simulink library "common_lib"  (R2021b)
settings: Solver=ode45  StartTime=0.0  StopTime=10.0  RelTol=1e-3
undefined symbols (not defined in the file or in its folder): ACCEL_PRE_MULT, C_C1GearNumbers, C_C1GearRatios, C_Calibration, C_DitherWaveform, C_GearOffset, C_GearRatioIn, C_GearRatioInverseOut, C_GearRatioOut, CLUTCH_INNER_LOOP_UPDATE_RATE, CONSTANT, DEGRADED_MODE_SIZE, Dem_EventStatusType, DiscIntNeverNeededParam, F_FAULT_ENUM, F_NOFAULT, F_OUTOFRANGE, F_RATELIMIT, FALSE, FMI14_SPECIAL_INSTRUCTIONS, FMI20_DATA_DRIFTED_HIGH, FMI21_DATA_DRIFTED_LOW, FMI29_RESERVED_FOR_SAE_ASSIGNMENT, FMI30_RESERVED_FOR_SAE_ASSIGNMENT, FMI31_CONDITION_EXISTS, FMI32_NO_FAULT, IC, k_accel, k_mean, LVDCU_OORH_FaultCntThd_C, MAX_UINT32, MEAN_PRE_MULT, NTriggers, QLTY_SIGNAL_FAILED, QLTY_SIGNAL_FULLY_FUNCTION, QLTY_SIGNAL_SUBSTITUTED_BY_1ST_CHOICE, QLTY_SIGNAL_SUBSTITUTED_BY_2ND_CHOICE, QLTY_SIGNAL_SUBSTITUTED_BY_3RD_CHOICE, QLTY_SIGNAL_SUBSTITUTED_BY_4TH_CHOICE, SAMPLE_TIME_100_mSec, SAMPLE_TIME_100_uSec, simin, T_TestPoint, TF_FALSE, TF_TRUE, TimeStep, TRUE, WORKSPACE_UPDATE_RATE, ZERO, Zero
libraries: $bdroot x120, simulink x27, simulink_extras x4, MBD_EPS_Local_Blockset x4
(part 7 of 10)

== system common_lib/OS/fcn_call generator ==
  note: This component is an atomic element used by the
      | schedule_morph script to build scheduler blocks
  note: Common Library::OS::Function Call Generator
  Enable : EnablePort  StatesWhenEnabling=reset  ZeroCross=off
  Function-Call Generator : simulink/Ports & Subsystems/Function-Call Generator  sample_time=-1  numberOfIterations=1  DisallowWideOutput=off
  Out : Outport  VectorParamsAs1DForOutWhenUnconnected=off
  wires:
  Function-Call Generator/1 -> Out/1

== system common_lib/OS/schedule counter ==
  note: This component is an atomic element used by the
      | schedule_morph script to build scheduler blocks
  note: Common Library::OS::Schedule Counter
  Constant2 : Constant  Value=int8(1)
  Constant3 : Constant  Value=int8(1)
  Constant4 : Constant  Value=FALSE
  Constant5 : Constant  Value=int8(1)
  Logical Operator : Logic  Operator=OR
  MinMax1 : MinMax  Inputs=2  InputSameDT=on  ZeroCross=off
  NTriggers : Constant  Value=NTriggers
  Relational Operator1 : RelationalOperator  Operator=>  ZeroCross=off  RndMeth=Nearest
  Sum : Sum  Inputs=++|  InputSameDT=on  OutDataTypeStr=Inherit: Same as first input
  Sum1 : Sum  Inputs=|-+  InputSameDT=on  OutDataTypeStr=Inherit: Same as first input
  Unit Delay : UnitDelay  InitialCondition=int8(1)  SampleTime=-1  HasFrameUpgradeWarning=on
  Unit Delay1 : UnitDelay  InitialCondition=TRUE  SampleTime=-1  HasFrameUpgradeWarning=on
  reset switch : Switch  Threshold=0.5  ZeroCross=off  InputSameDT=on
  Counter : Outport  VectorParamsAs1DForOutWhenUnconnected=off
  wires:
  Constant5/1 -> Sum1/1
  Sum/1 -> MinMax1/2
  NTriggers/1 -> Sum1/2, MinMax1/1
  Sum1/1 -> Relational Operator1/2
  Relational Operator1/1 -> Logical Operator/1
  Constant3/1 -> reset switch/1
  MinMax1/1 -> reset switch/3
  Constant2/1 -> Sum/2
  Constant4/1 -> Unit Delay1/1
  Unit Delay1/1 -> Logical Operator/2
  Logical Operator/1 -> reset switch/2
  Unit Delay/1 -> Relational Operator1/1, Sum/1
  reset switch/1 -> Unit Delay/1, Counter/1

== system common_lib/OS/sequence generator ==
  note: This component is an atomic element used by the
      | schedule_morph script to build scheduler blocks
  note: Common Library::OS::Sequence Generator
  In : Inport
  Constant9 : Constant  Value=int8(1)
  Function-Call Generator : simulink/Ports & Subsystems/Function-Call Generator  sample_time=-1  numberOfIterations=1  DisallowWideOutput=off
  Sum1 : Sum  Inputs=|++  InputSameDT=on  OutDataTypeStr=Inherit: Same as first input
  Trigger : Outport  VectorParamsAs1DForOutWhenUnconnected=off
  Out : Outport  Port=2  VectorParamsAs1DForOutWhenUnconnected=off
  wires:
  Function-Call Generator/1 -> Trigger/1
  Constant9/1 -> Sum1/2
  In/1 -> Sum1/1
  Sum1/1 -> Out/1

== system common_lib/SCond/Gain and Offset (in) ==
  note: Common Library::Signal Conditioning::Gain and Offset (in)
  input : Inport
  gain : Inport  Port=2
  offset : Inport  Port=3
  InputConversion : DataTypeConversion  OutDataTypeStr=single  RndMeth=Zero
  InputConversion1 : DataTypeConversion  OutDataTypeStr=single  RndMeth=Zero
  InputConversion2 : DataTypeConversion  OutDataTypeStr=single  RndMeth=Zero
  OutputConversion : DataTypeConversion  OutDataTypeStr=single  RndMeth=Zero
  Product : Product  InputSameDT=on  OutDataTypeStr=Inherit: Same as first input
  Sum : Sum  Inputs=|+-  InputSameDT=on  OutDataTypeStr=Inherit: Same as first input
  output : Outport  VectorParamsAs1DForOutWhenUnconnected=off
  wires:
  OutputConversion/1 -> output/1
  input/1 -> InputConversion/1
  gain/1 -> InputConversion1/1
  Product/1 -> Sum/1
  offset/1 -> InputConversion2/1
  Sum/1 -> OutputConversion/1
  InputConversion/1 -> Product/1
  InputConversion1/1 -> Product/2
  InputConversion2/1 -> Sum/2

== system common_lib/SCond/Gain and Offset (out) ==
  note: Common Library::Signal Conditioning::Gain and Offset (out)
  input : Inport
  gain : Inport  Port=2
  offset : Inport  Port=3
  InputConversion : DataTypeConversion  OutDataTypeStr=single  RndMeth=Zero
  InputConversion1 : DataTypeConversion  OutDataTypeStr=single  RndMeth=Zero
  InputConversion2 : DataTypeConversion  OutDataTypeStr=single  RndMeth=Zero
  OutputConversion : DataTypeConversion  OutDataTypeStr=single  RndMeth=Zero
  Product : Product  Inputs=*/  InputSameDT=on  OutDataTypeStr=Inherit: Same as first input
  Sum : Sum  Inputs=|++  InputSameDT=on  OutDataTypeStr=Inherit: Same as first input
  output : Outport  VectorParamsAs1DForOutWhenUnconnected=off
  wires:
  Sum/1 -> Product/1
  input/1 -> InputConversion/1
  OutputConversion/1 -> output/1
  offset/1 -> InputConversion1/1
  gain/1 -> InputConversion2/1
  Product/1 -> OutputConversion/1
  InputConversion/1 -> Sum/1
  InputConversion1/1 -> Sum/2
  InputConversion2/1 -> Product/2

== system common_lib/SCond/Membership Function ==
  x : Inport
  Compare1 : RelationalOperator  Operator=<=  ZeroCross=off  RndMeth=Nearest  InputSameDT=on
  MinMax : MinMax  Function=max  Inputs=2  InputSameDT=on  SaturateOnIntegerOverflow=on  ZeroCross=off
  Product2 : Product  Inputs=**  OutDataTypeStr=Inherit: Same as first input
  Sum1 : Sum  Inputs=|++  InputSameDT=on  OutDataTypeStr=Inherit: Same as first input
  Sum2 : Sum  Inputs=-+|  InputSameDT=on  OutDataTypeStr=Inherit: Same as first input
  Switch1 : Switch  Criteria=u2 ~= 0  Threshold=0.5  ZeroCross=off  InputSameDT=on
  TRUE1 : Constant  Value=SlopeLow
  TRUE3 : Constant  Value=Peak
  TRUE4 : Constant  Value=One
  TRUE5 : Constant  Value=Zero
  TRUE6 : Constant  Value=SlopeHigh
  TRUE7 : Constant  Value=Peak
  mu(x) : Outport  VectorParamsAs1DForOutWhenUnconnected=off
  wires:
  Sum1/1 -> MinMax/2
  Switch1/1 -> Product2/2
  Product2/1 -> Sum1/1
  TRUE3/1 -> Compare1/2
  Compare1/1 -> Switch1/2
  TRUE6/1 -> Switch1/3
  TRUE1/1 -> Switch1/1
  Sum2/1 -> Product2/1
  TRUE7/1 -> Sum2/1
  x/1 -> Compare1/1, Sum2/2
  TRUE4/1 -> Sum1/2
  TRUE5/1 -> MinMax/1
  MinMax/1 -> mu(x)/1

== system common_lib/SCond/Test Override Gain and Offset (in) ==
  note: This block  accepts the Inputsignal, gain, offset, and override flag
      |
      | This block does the  functionality of Y =mX+b
      | Where  Y  = Output
      |               m = Override_Gain
      |               X  = Input
      |               b = Override_Offset
  note: Common Library::Signal Override::Gain , Offset ,Override flag
  Input : Inport
  Override_Gain : Inport  Port=2
  Override_Offset : Inport  Port=3
  Override_Flag : Inport  Port=4
  InputConversion : DataTypeConversion  OutDataTypeStr=single  RndMeth=Zero
  InputConversion1 : DataTypeConversion  OutDataTypeStr=single  RndMeth=Zero
  InputConversion2 : DataTypeConversion  OutDataTypeStr=single  RndMeth=Zero
  OutputConversion : DataTypeConversion  OutDataTypeStr=single  RndMeth=Zero
  Product : Product  InputSameDT=on  OutDataTypeStr=Inherit: Same as first input
  Sum : Sum  Inputs=|++  InputSameDT=on  OutDataTypeStr=Inherit: Same as first input
  Switch : Switch  Threshold=0.5  ZeroCross=off
  Output : Outport  VectorParamsAs1DForOutWhenUnconnected=off
  wires:
  InputConversion2/1 -> Sum/2
  InputConversion1/1 -> Product/2
  InputConversion/1 -> Product/1
  Sum/1 -> OutputConversion/1
  Product/1 -> Sum/1
  Input/1 -> InputConversion/1, Switch/3
  Switch/1 -> Output/1
  Override_Offset/1 -> InputConversion2/1
  Override_Flag/1 -> Switch/2
  Override_Gain/1 -> InputConversion1/1
  OutputConversion/1 -> Switch/1

== system common_lib/SCond/ramp to zero ==
  note: Common Library::Signal Conditioning::Ramp to Zero
  note: factor is zero at zero speed
      | factor is 1 or -1 if the abs value of spd is > limit
      | factor is linear between 1 and-1 if the abs value of spd < limit
      | the sign of factor is the same as the sign of speed
  speed : Inport
  limit : Inport  Port=2
  Abs : Abs  ZeroCross=off
  Constant : Constant  Value=One
  Constant1 : Constant  Value=MinusOne
  Constant2 : Constant  Value=Zero
  Product1 : Product  Inputs=*/  InputSameDT=on  OutDataTypeStr=Inherit: Same as first input
  Relational Operator : RelationalOperator  Operator=<  ZeroCross=off  RndMeth=Nearest  InputSameDT=on
  Relational Operator1 : RelationalOperator  ZeroCross=off  RndMeth=Nearest  InputSameDT=on
  Switch : Switch  Threshold=0.5  ZeroCross=off  InputSameDT=on
  Switch1 : Switch  Threshold=0.5  ZeroCross=off  InputSameDT=on
  factor : Outport  VectorParamsAs1DForOutWhenUnconnected=off
  wires:
  speed/1 -> Abs/1, Relational Operator1/1, Product1/1
  Abs/1 -> Relational Operator/1
  limit/1 -> Product1/2, Relational Operator/2
  Product1/1 -> Switch/1
  Relational Operator/1 -> Switch/2
  Constant/1 -> Switch1/1
  Switch/1 -> factor/1
  Constant1/1 -> Switch1/3
  Constant2/1 -> Relational Operator1/2
  Relational Operator1/1 -> Switch1/2
  Switch1/1 -> Switch/3

== system common_lib/Signal Conditioning/2nd Order Butterworth Filter ==
  note: DO NOT CHANGE 2.0 DAMPING CONSTANT
  note: This is a 2nd order butterworth filter.
      | When Disable is true the raw value is
      | passed through.
  note: The Integrator blocks in common_lib don't work as well
      | for this filter.
  Input : Inport
  CutoffFreq : Inport  Port=2
  Reset : Inport  Port=3
  ClampAboveZero : $bdroot/Misc/ClampAboveZero  Tol=single(0.001)
      settings: AttributesFormatString=tol=%<Tol>
  Constant1 : Constant  Value=single(0.0)  SampleTime=-1
  Constant2 : Constant  Value=single(2.0)  SampleTime=-1
  Constant3 : Constant  Value=TSAMP  SampleTime=-1
  Constant4 : Constant  Value=single(1.0)  SampleTime=-1
  Data Type Conversion : DataTypeConversion  OutDataTypeStr=single  RndMeth=Zero
  Divide : Product  Inputs=***
  Divide1 : Product  Inputs=***
  Divide2 : Product  Inputs=*/
  ForwardEulerIntergrator1 : MBD_EPS_Local_Blockset/Integrators/ForwardEulerIntergrator  IC=single(0.0)  TSAMP=TSAMP
  ForwardEulerIntergrator2 : MBD_EPS_Local_Blockset/Integrators/ForwardEulerIntergrator  IC=IC  TSAMP=TSAMP
  MinMax : MinMax  Inputs=2  InputSameDT=on  ZeroCross=off
  Sum : Sum  Inputs=|+-
  Sum1 : Sum  Inputs=|+-
  PtmShiftMotorTorqueCmd : Outport  VectorParamsAs1DForOutWhenUnconnected=off
  wires:
  Input/1 -> Sum/1, ForwardEulerIntergrator2/2
  Reset/1 -> ForwardEulerIntergrator2/3, ForwardEulerIntergrator1/3
  ForwardEulerIntergrator1/1 -> Divide1/3, ForwardEulerIntergrator2/1
  Sum1/1 -> ForwardEulerIntergrator1/1
  Divide1/1 -> Sum1/2
  Constant2/1 -> Divide1/2
  Sum/1 -> Divide/1
  ForwardEulerIntergrator2/1 -> PtmShiftMotorTorqueCmd/1, Sum/2
  Divide/1 -> Sum1/1
  Constant1/1 -> ForwardEulerIntergrator1/2
  CutoffFreq/1 -> MinMax/1
  Constant3/1 -> Data Type Conversion/1
  Constant4/1 -> Divide2/1
  Data Type Conversion/1 -> ClampAboveZero/1
  ClampAboveZero/1 -> Divide2/2
  Divide2/1 -> MinMax/2
  MinMax/1 -> [ProtectedCutoffFreq]
  [ProtectedCutoffFreq] -> Divide1/1, Divide/3, Divide/2

== system common_lib/Signal Conditioning/AnalogChecking ==
  in : Inport  OutDataTypeStr=Bus: BO_InputSignal
  u_lim : Inport  Port=2
  l_lim : Inport  Port=3
  r_lim : Inport  Port=4
  tau : Inport  Port=5
  overide : Inport  Port=6
  overide_value : Inport  Port=7
  Bitwise Operator : simulink/Logic and Bit Operations/Bitwise Operator  logicop=OR  UseBitMask=off  NumInputPorts=3  BitMask=bin2dec('11011001')  BitMaskRealWorld=Stored Integer
  Bus Creator2 : BusCreator  Inputs=2  OutDataTypeStr=Bus: BO_InputSignal
  Bus Selector1 : BusSelector  OutputSignals=value,FMI
  C_Calibration1 : Constant  Value=F_OUTOFRANGE
  C_Calibration2 : Constant  Value=F_NOFAULT
  C_Calibration3 : Constant  Value=false
  C_Calibration4 : Constant  Value=F_RATELIMIT
  C_Calibration5 : Constant  Value=F_NOFAULT
  C_Calibration6 : Constant  Value=false
  C_Calibration7 : Constant  Value=F_NOFAULT
  C_Calibration8 : Constant  Value=false
  Fltr_wR : $bdroot/Fltrs/Fltr_wR  TimeStep=TimeStep
  Logical Operator : Logic  Operator=OR
  OOR Fault Detection : $bdroot/Diag/OOR Fault Detection  InitialValue=0
  Rate Limit Fault Detection : $bdroot/Diag/Rate Limit Fault Detection  IC=0  TimeStep=TimeStep
  Relational Operator : RelationalOperator  Operator=~=  OutDataTypeStr=boolean  ZeroCross=off  RndMeth=Nearest
  Switch : Switch  Threshold=0.5  ZeroCross=off
  Switch1 : Switch  Threshold=0.5  ZeroCross=off
  Switch2 : Switch  Threshold=0.5  ZeroCross=off
  Unit Delay : UnitDelay  InitialCondition=true  SampleTime=-1  HasFrameUpgradeWarning=on
      settings: AttributesFormatString=ic=%<X0>
  out : Outport  VectorParamsAs1DForOutWhenUnconnected=off
  wires:
  Relational Operator/1 -> Logical Operator/2
  Logical Operator/1 -> Fltr_wR/4
  Unit Delay/1 -> Logical Operator/1
  C_Calibration8/1 -> Unit Delay/1
  Bus Selector1/1 -> OOR Fault Detection/1  "<value>"
  C_Calibration6/1 -> OOR Fault Detection/4
  in/1 -> Bus Selector1/1
  OOR Fault Detection/1 -> Rate Limit Fault Detection/1
  u_lim/1 -> OOR Fault Detection/2
  l_lim/1 -> OOR Fault Detection/3
  Bus Selector1/2 -> Bitwise Operator/3  "<FMI>"
  OOR Fault Detection/2 -> Switch/2
  Switch/1 -> Bitwise Operator/2
  C_Calibration1/1 -> Switch/1
  C_Calibration2/1 -> Switch/3
  Bus Creator2/1 -> out/1
  Rate Limit Fault Detection/1 -> Fltr_wR/3, Fltr_wR/1
  r_lim/1 -> Rate Limit Fault Detection/2
  C_Calibration3/1 -> Rate Limit Fault Detection/3
  Rate Limit Fault Detection/2 -> Switch1/2
  C_Calibration4/1 -> Switch1/1
  C_Calibration5/1 -> Switch1/3
  Switch1/1 -> Bitwise Operator/1
  Bitwise Operator/1 -> Bus Creator2/2, Relational Operator/2  "FMI"
  tau/1 -> Fltr_wR/2
  C_Calibration7/1 -> Relational Operator/1
  overide/1 -> Switch2/2
  overide_value/1 -> Switch2/1
  Fltr_wR/1 -> Switch2/3  "value"
  Switch2/1 -> Bus Creator2/1  "value"

== system common_lib/Signal Conditioning/DitherSaturation ==
  signal_in : Inport
  max_signal_amp : Inport  Port=2
  dither_amplitude : Inport  Port=3
  dither_in : Inport  Port=4
  Constant1 : Constant  Value=0  OutDataTypeStr=single
  Constant2 : Constant  Value=single(1)
  Constant3 : Constant  Value=eps  OutDataTypeStr=single
  MinMax1 : MinMax  Inputs=2
  MinMax2 : MinMax  Inputs=2
  MinMax3 : MinMax  Function=max  Inputs=2
  MinMax4 : MinMax  Inputs=2
  MinMax5 : MinMax  Function=max  Inputs=2
  Product : Product  RndMeth=Zero
  Product1 : Product  RndMeth=Zero
  Product2 : Product  Inputs=/*  RndMeth=Zero
  Product3 : Product  Inputs=/*  RndMeth=Zero
  Sum : Sum  Inputs=|-+
  Sum1 : Sum  Inputs=|++
  out : Outport  VectorParamsAs1DForOutWhenUnconnected=off
  wires:
  Constant1/1 -> MinMax5/2
  signal_in/1 -> MinMax5/1
  MinMax5/1 -> MinMax4/2
  MinMax4/1 -> Product2/2, Sum/1, Sum1/2
  Product1/1 -> Sum1/1
  Sum1/1 -> out/1
  dither_in/1 -> Product/1
  MinMax3/1 -> Product2/1, Product3/1
  Constant3/1 -> MinMax3/2
  Product/1 -> Product1/1
  Product3/1 -> MinMax1/2
  Sum/1 -> Product3/2
  Product2/1 -> MinMax1/1
  MinMax2/1 -> Product1/2
  MinMax1/1 -> MinMax2/2
  Constant2/1 -> MinMax2/1
  max_signal_amp/1 -> MinMax4/1, Sum/2
  dither_amplitude/1 -> Product/2, MinMax3/1

== system common_lib/Signal Conditioning/DitherSaturation1 ==
  signal_in : Inport
  max_signal_amp : Inport  Port=2
  dither_amplitude : Inport  Port=3
  dither_in : Inport  Port=4
  Constant1 : Constant  Value=0  OutDataTypeStr=single
  Constant2 : Constant  Value=single(1)
  Constant3 : Constant  Value=eps  OutDataTypeStr=single
  MinMax1 : MinMax  Inputs=2
  MinMax2 : MinMax  Inputs=2
  MinMax3 : MinMax  Function=max  Inputs=2
  MinMax4 : MinMax  Inputs=2
  MinMax5 : MinMax  Function=max  Inputs=2
  Product : Product  RndMeth=Zero
  Product1 : Product  RndMeth=Zero
  Product2 : Product  Inputs=/*  RndMeth=Zero
  Product3 : Product  Inputs=/*  RndMeth=Zero
  Sum : Sum  Inputs=|-+
  Sum1 : Sum  Inputs=|++
  out : Outport  VectorParamsAs1DForOutWhenUnconnected=off
  wires:
  Constant1/1 -> MinMax5/2
  signal_in/1 -> MinMax5/1
  MinMax5/1 -> MinMax4/2
  MinMax4/1 -> Product2/2, Sum/1, Sum1/2
  Product1/1 -> Sum1/1
  Sum1/1 -> out/1
  dither_in/1 -> Product/1
  MinMax3/1 -> Product2/1, Product3/1
  Constant3/1 -> MinMax3/2
  Product/1 -> Product1/1
  Product3/1 -> MinMax1/2
  Sum/1 -> Product3/2
  Product2/1 -> MinMax1/1
  MinMax2/1 -> Product1/2
  MinMax1/1 -> MinMax2/2
  Constant2/1 -> MinMax2/1
  max_signal_amp/1 -> MinMax4/1, Sum/2
  dither_amplitude/1 -> Product/2, MinMax3/1

== system common_lib/Signal Conditioning/HydValveDither ==
  freq_hz : Inport
  CalculateActualFreq : Subsystem
  Constant : Constant  Value=single(ts)
  Constant4 : Constant  Value=single(0)
  Switch : Switch  Criteria=u2 > Threshold
  TableBasedSignalGen : Subsystem
  out : Outport  VectorParamsAs1DForOutWhenUnconnected=off
  realized_freq : Outport  Port=2  VectorParamsAs1DForOutWhenUnconnected=off
  wires:
  Constant4/1 -> Switch/3
  TableBasedSignalGen/1(out) -> Switch/1
  freq_hz/1 -> CalculateActualFreq/1(desired_freqency_hz), Switch/2
  CalculateActualFreq/2(sample_times_per_cycle) -> TableBasedSignalGen/1(sample_times_per_cycle)
  CalculateActualFreq/1(realized_freq) -> realized_freq/1
  Constant/1 -> CalculateActualFreq/2(sample_time)
  Switch/1 -> out/1

== system common_lib/Signal Conditioning/Normalized Variable Tanh Curve ==
  note: Time Input
  note: This block handles a changing Target Time
  note: ******************************************************************************************************************************************************
      | UNPUBLISHED AND CONFIDENTIAL. COPYRIGHT EATON CORPORATION, CREATED 2002, ALL RIGHTS RESERVED.
      | NOT TO BE REPRODUCED, DISSEMINATED, TRANSFERRED OR USED WITHOUT THE PRIOR WRITTEN CONSENT OF
      | EATON CORPORATION.
      | ******************************************************************************************************************************************************
  RampTime : Inport
  Reset : Inport  Port=2
  ClampAboveZero : $bdroot/Misc/ClampAboveZero  Tol=single(0.001)
      settings: AttributesFormatString=tol=%<Tol>
  Constant12 : Constant  Value=single(1000)  SampleTime=-1
  Constant13 : Constant  Value=single(-1000)  SampleTime=-1
  Constant3 : Constant  Value=TimeStep  SampleTime=-1
  Constant7 : Constant  Value=single(0)  SampleTime=-1
  Constant8 : Constant  Value=single(-1000)  SampleTime=-1
  Constant9 : Constant  Value=single(0.0)  SampleTime=-1
  Data Type Conversion : DataTypeConversion  OutDataTypeStr=single  RndMeth=Zero
  Lookup Table Tanh : Lookup  InputValues=single([0 0.125 0.25 0.375 0.5 0.625 0.75 0.875 1])  Table=single([0 0.04745 0.1192 0.26895 0.5 0.73105 0.8808 0.95255 1])  LookUpMeth=Interpolation-Use End Values
  Product1 : Product  Inputs=*/  OutDataTypeStr=Inherit: Same as first input
  Sum1 : Sum  Inputs=|++
  Switch : Switch  Threshold=0.5  ZeroCross=off
  Trajectory : MBD_EPS_Local_Blockset/Trajectory Modification/Trajectory  TimeStep=TimeStep  wn=single(30)  damping=single(.8)
  Unit Delay : UnitDelay  InitialCondition=single(0.0)  SampleTime=-1  HasFrameUpgradeWarning=on
      settings: AttributesFormatString=ic=%<X0>
  Out : Outport  VectorParamsAs1DForOutWhenUnconnected=off
  wires:
  Product1/1 -> Lookup Table Tanh/1
  Unit Delay/1 -> Sum1/2
  Constant3/1 -> Data Type Conversion/1
  Constant7/1 -> Trajectory/2
  Lookup Table Tanh/1 -> Out/1
  Trajectory/1 -> ClampAboveZero/1
  RampTime/1 -> Trajectory/1
  Constant8/1 -> Trajectory/3
  Constant12/1 -> Trajectory/4
  Constant13/1 -> Trajectory/5
  Reset/1 -> Switch/2, Trajectory/6
  Constant9/1 -> Switch/1
  Sum1/1 -> Switch/3
  Switch/1 -> Unit Delay/1, Product1/1
  ClampAboveZero/1 -> Product1/2
  Data Type Conversion/1 -> Sum1/1

== system common_lib/Signal Conditioning/Obsolete Signal Conditioning ==
  note: Obsolete Signal Conditioning
  BooleanToTernary : Subsystem
      mask Display:
      | patch([0.3 0.3 0.7 0.7], [0.4 0.6 0.6 0.4], [255/255 127/255 255/255]);
      | disp('Boolean to Ternary')
  Ternary To Boolean (Default False) : Subsystem
      mask Display:
      | patch([0.3 0.3 0.7 0.7], [0.4 0.6 0.6 0.4], [255/255 127/255 255/255]);
      | disp('Ternary To Boolean\n(Default False)')
  Ternary To Boolean (Default True) : Subsystem
      mask Display:
      | patch([0.3 0.3 0.7 0.7], [0.4 0.6 0.6 0.4], [255/255 127/255 255/255]);
      | disp('Ternary To Boolean \n (Default True)')

== system common_lib/Signal Conditioning/OffsetAndGain ==
  input : Inport
  gain : Inport  Port=2
  offset : Inport  Port=3
  Data Type Conversion : DataTypeConversion  OutDataTypeStr=single
  Data Type Conversion1 : DataTypeConversion  OutDataTypeStr=single
  Data Type Conversion2 : DataTypeConversion  OutDataTypeStr=single
  Product : Product  InputSameDT=on  OutDataTypeStr=Inherit: Same as first input
  Sum : Sum  InputSameDT=on  OutDataTypeStr=Inherit: Same as first input
  output : Outport  VectorParamsAs1DForOutWhenUnconnected=off
  wires:
  Data Type Conversion2/1 -> Product/2
  Data Type Conversion1/1 -> Sum/2
  Data Type Conversion/1 -> Sum/1
  Sum/1 -> Product/1
  Product/1 -> output/1
  offset/1 -> Data Type Conversion/1
  gain/1 -> Data Type Conversion2/1
  input/1 -> Data Type Conversion1/1

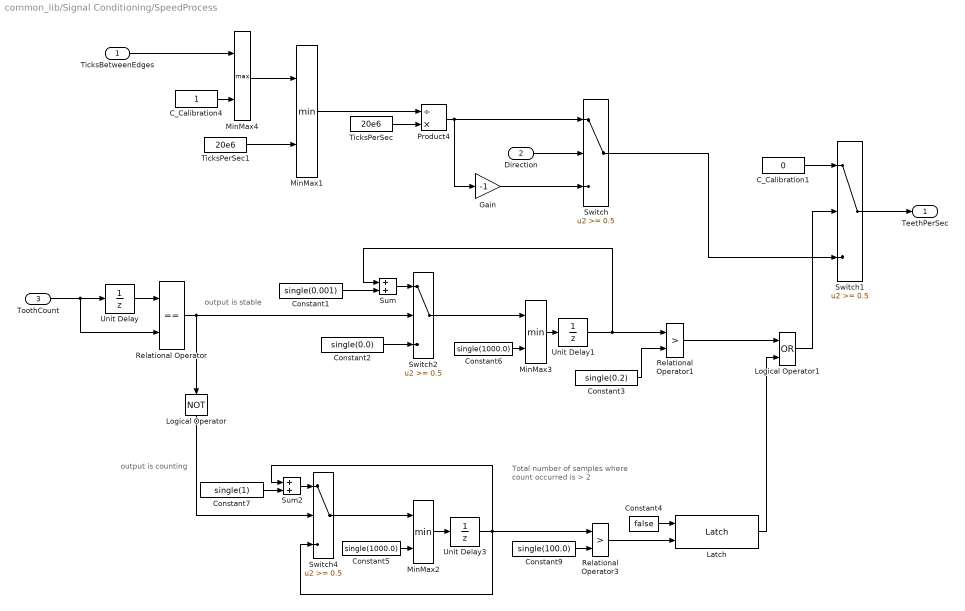
== system common_lib/Signal Conditioning/SpeedProcess ==
  note: output is stable
  note: output is counting
  note: Total number of samples where
      | count occurred is > 2
  TicksBetweenEdges : Inport
  Direction : Inport  Port=2
  ToothCount : Inport  Port=3
  C_Calibration1 : Constant  Value=0
  C_Calibration4 : Constant
  Constant1 : Constant  Value=single(0.001)
  Constant2 : Constant  Value=single(0.0)
  Constant3 : Constant  Value=single(0.2)
  Constant4 : Constant  Value=false
  Constant5 : Constant  Value=single(1000.0)
  Constant6 : Constant  Value=single(1000.0)
  Constant7 : Constant  Value=single(1)
  Constant9 : Constant  Value=single(100.0)
  Gain : Gain  Gain=-1
  Latch : $bdroot/Misc/Latch  IC=true
  Logical Operator : Logic  Operator=NOT
  Logical Operator1 : Logic  Operator=OR  AllPortsSameDT=off
  MinMax1 : MinMax  Inputs=2  InputSameDT=on  ZeroCross=off
  MinMax2 : MinMax  Inputs=2  InputSameDT=on  ZeroCross=off
  MinMax3 : MinMax  Inputs=2  InputSameDT=on  ZeroCross=off
  MinMax4 : MinMax  Function=max  Inputs=2  InputSameDT=on  ZeroCross=off
  Product4 : Product  Inputs=/*  RndMeth=Zero
  Relational Operator : RelationalOperator  Operator===  OutDataTypeStr=boolean  RndMeth=Nearest
  Relational Operator1 : RelationalOperator  Operator=>  ZeroCross=off  RndMeth=Nearest
  Relational Operator3 : RelationalOperator  Operator=>  ZeroCross=off  RndMeth=Nearest
  Sum : Sum
  Sum2 : Sum
  Switch{,1..2,4} (4 alike) : Switch  Threshold=0.5  ZeroCross=off
  TicksPerSec : Constant  Value=20e6
  TicksPerSec1 : Constant  Value=20e6
  Unit Delay : UnitDelay  SampleTime=0.001  HasFrameUpgradeWarning=on
  Unit Delay1 : UnitDelay  InitialCondition=single(0)  SampleTime=0.001  HasFrameUpgradeWarning=on
  Unit Delay3 : UnitDelay  InitialCondition=single(0)  SampleTime=0.001  HasFrameUpgradeWarning=on
  TeethPerSec : Outport  VectorParamsAs1DForOutWhenUnconnected=off
  wires:
  Constant3/1 -> Relational Operator1/2
  Constant2/1 -> Switch2/3
  Unit Delay1/1 -> Relational Operator1/1, Sum/1
  MinMax1/1 -> Product4/1
  TicksPerSec1/1 -> MinMax1/2
  MinMax4/1 -> MinMax1/1
  Switch1/1 -> TeethPerSec/1
  TicksPerSec/1 -> Product4/2
  TicksBetweenEdges/1 -> MinMax4/1
  Direction/1 -> Switch/2
  Gain/1 -> Switch/3
  Product4/1 -> Gain/1, Switch/1
  ToothCount/1 -> Unit Delay/1, Relational Operator/2
  C_Calibration4/1 -> MinMax4/2
  Unit Delay/1 -> Relational Operator/1
  Sum/1 -> Switch2/1
  Constant1/1 -> Sum/2
  Relational Operator/1 -> Switch2/2, Logical Operator/1
  C_Calibration1/1 -> Switch1/1
  Switch/1 -> Switch1/3
  Logical Operator/1 -> Switch4/2
  Constant9/1 -> Relational Operator3/2
  Unit Delay3/1 -> Sum2/1, Switch4/3, Relational Operator3/1
  Sum2/1 -> Switch4/1
  Constant7/1 -> Sum2/2
  Latch/1 -> Logical Operator1/2
  Relational Operator3/1 -> Latch/2
  Constant4/1 -> Latch/1
  Relational Operator1/1 -> Logical Operator1/1
  Logical Operator1/1 -> Switch1/2
  MinMax2/1 -> Unit Delay3/1
  Switch4/1 -> MinMax2/1
  Constant5/1 -> MinMax2/2
  MinMax3/1 -> Unit Delay1/1
  Constant6/1 -> MinMax3/2
  Switch2/1 -> MinMax3/1

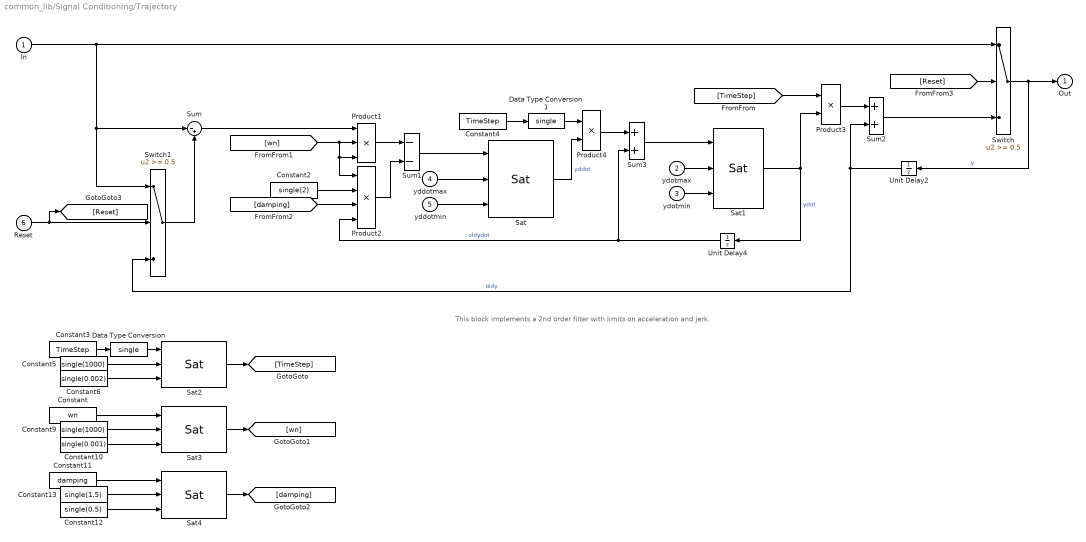
== system common_lib/Signal Conditioning/Trajectory ==
  note: This block implements a 2nd order filter with limits on acceleration and jerk.
  In : Inport
  ydotmax : Inport  Port=2
  ydotmin : Inport  Port=3
  yddotmax : Inport  Port=4
  yddotmin : Inport  Port=5
  Reset : Inport  Port=6
  Constant : Constant  Value=wn  SampleTime=-1
  Constant10 : Constant  Value=single(0.001)  SampleTime=-1
  Constant11 : Constant  Value=damping  SampleTime=-1
  Constant12 : Constant  Value=single(0.5)  SampleTime=-1
  Constant13 : Constant  Value=single(1.5)  SampleTime=-1
  Constant2 : Constant  Value=single(2)  SampleTime=-1
  Constant3 : Constant  Value=TimeStep  SampleTime=-1
  Constant4 : Constant  Value=TimeStep  SampleTime=-1
  Constant5 : Constant  Value=single(1000)  SampleTime=-1
  Constant6 : Constant  Value=single(0.002)  SampleTime=-1
  Constant9 : Constant  Value=single(1000)  SampleTime=-1
  Data Type Conversion : DataTypeConversion  OutDataTypeStr=single  RndMeth=Zero
  Data Type Conversion1 : DataTypeConversion  OutDataTypeStr=single  RndMeth=Zero
  Product1 : Product  Inputs=3  OutDataTypeStr=Inherit: Same as first input
  Product2 : Product  Inputs=4  OutDataTypeStr=Inherit: Same as first input
  Product3 : Product  OutDataTypeStr=Inherit: Same as first input
  Product4 : Product  OutDataTypeStr=Inherit: Same as first input
  Sat{,1..4} (5 alike) : $bdroot/Slink/Sat
  Sum : Sum  Inputs=|-+
  Sum1 : Sum  Inputs=--
  Sum2 : Sum
  Sum3 : Sum
  Switch : Switch  Threshold=0.5  ZeroCross=off
  Switch1 : Switch  Threshold=0.5  ZeroCross=off
  Unit Delay2 : UnitDelay  InitialCondition=single(0.0)  SampleTime=-1  HasFrameUpgradeWarning=on
      settings: AttributesFormatString=ic=%<X0>
  Unit Delay4 : UnitDelay  InitialCondition=single(0.0)  SampleTime=-1  HasFrameUpgradeWarning=on
      settings: AttributesFormatString=ic=%<X0>
  Out : Outport  VectorParamsAs1DForOutWhenUnconnected=off
  wires:
  In/1 -> Switch/1, Switch1/1, Sum/1
  Sum/1 -> Product1/1
  Product2/1 -> Sum1/2
  Product1/1 -> Sum1/1
  Product3/1 -> Sum2/1
  Constant4/1 -> Data Type Conversion1/1
  Product4/1 -> Sum3/1
  Sum3/1 -> Sat1/1
  Constant2/1 -> Product2/2
  Sum1/1 -> Sat/1
  yddotmax/1 -> Sat/2
  yddotmin/1 -> Sat/3
  Sat/1 -> Product4/2  "yddot"
  ydotmax/1 -> Sat1/2
  Sat1/1 -> Unit Delay4/1, Product3/2  "ydot"
  Switch/1 -> Out/1, Unit Delay2/1  "y"
  Sum2/1 -> Switch/3
  Unit Delay2/1 -> Sum2/2, Switch1/3  "oldy"
  Unit Delay4/1 -> Sum3/2, Product2/4  "oldydot"
  Switch1/1 -> Sum/2
  ydotmin/1 -> Sat1/3
  Constant3/1 -> Data Type Conversion/1
  Constant5/1 -> Sat2/2
  Constant6/1 -> Sat2/3
  Sat2/1 -> [TimeStep]
  [TimeStep] -> Product3/1
  Constant/1 -> Sat3/1
  Constant9/1 -> Sat3/2
  Constant10/1 -> Sat3/3
  Sat3/1 -> [wn]
  [wn] -> Product1/2, Product1/3, Product2/1
  Constant11/1 -> Sat4/1
  Constant13/1 -> Sat4/2
  Constant12/1 -> Sat4/3
  Sat4/1 -> [damping]
  [damping] -> Product2/3
  Reset/1 -> Switch1/2, [Reset]
  [Reset] -> Switch/2
  Data Type Conversion/1 -> Sat2/1
  Data Type Conversion1/1 -> Product4/1

== system common_lib/Signal Conditioning/Variable Tanh Curve ==
  note: ******************************************************************************************************************************************************
      | UNPUBLISHED AND CONFIDENTIAL. COPYRIGHT EATON CORPORATION, CREATED 2002, ALL RIGHTS RESERVED.
      | NOT TO BE REPRODUCED, DISSEMINATED, TRANSFERRED OR USED WITHOUT THE PRIOR WRITTEN CONSENT OF
      | EATON CORPORATION.
      | ******************************************************************************************************************************************************
  StartValue : Inport
  FinalValue : Inport  Port=2
  RampTime : Inport  Port=3
  Reset : Inport  Port=4
  Constant1 : Constant  Value=single(0.01)  SampleTime=-1
  Constant10 : Constant  Value=single(1.0)  SampleTime=-1
  Normalized Variable Tanh Curve : MBD_EPS_Local_Blockset/Trajectory Modification/Normalized Variable Tanh Curve  TimeStep=TimeStep
  Product2 : Product  OutDataTypeStr=Inherit: Same as first input
  Relational Operator : RelationalOperator  Operator=<=  ZeroCross=off  RndMeth=Nearest
  Sum2 : Sum  Inputs=|+-
  Sum5 : Sum  Inputs=|+-
  Sum6 : Sum  Inputs=+-|
  Switch : Switch  Threshold=0.5  ZeroCross=off
  Unit Delay1 : UnitDelay  InitialCondition=single(0.0)  SampleTime=-1  HasFrameUpgradeWarning=on
      settings: AttributesFormatString=ic=%<X0>
  Out : Outport  VectorParamsAs1DForOutWhenUnconnected=off
  RampComplete : Outport  Port=2  VectorParamsAs1DForOutWhenUnconnected=off
  wires:
  RampTime/1 -> Normalized Variable Tanh Curve/1
  FinalValue/1 -> Sum5/1, Sum6/1
  StartValue/1 -> Switch/1
  Switch/1 -> Unit Delay1/1, Sum6/2
  Unit Delay1/1 -> Switch/3
  Constant10/1 -> Sum2/1
  Normalized Variable Tanh Curve/1 -> Sum2/2
  Sum6/1 -> Product2/1
  Sum2/1 -> Product2/2, Relational Operator/1
  Product2/1 -> Sum5/2
  Sum5/1 -> Out/1
  Constant1/1 -> Relational Operator/2
  Relational Operator/1 -> RampComplete/1
  Reset/1 -> Switch/2, Normalized Variable Tanh Curve/2

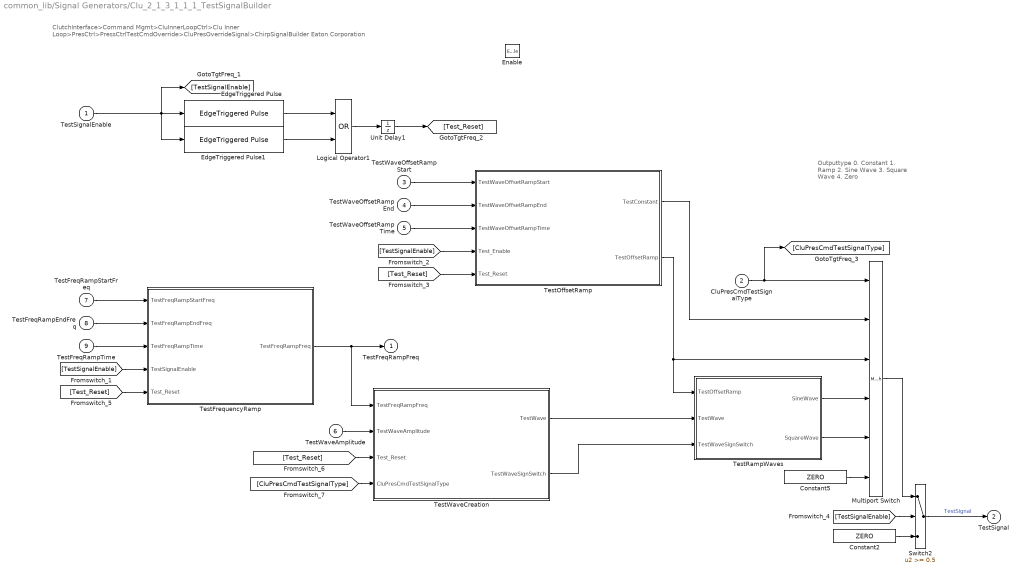
== system common_lib/Signal Generators/Clu_2_1_3_1_1_1_TestSignalBuilder ==
  note: ClutchInterface>Command Mgmt>CluInnerLoopCtrl>Clu Inner Loop>PresCtrl>PressCtrlTestCmdOverride>CluPresOverrideSignal>ChirpSignalBuilder
      | Eaton Corporation
  note: Outputtype
      | 0. Constant
      | 1. Ramp
      | 2. Sine Wave
      | 3. Square Wave
      | 4. Zero
  TestSignalEnable : Inport
  CluPresCmdTestSignalType : Inport  Port=2
  TestWaveOffsetRampStart : Inport  Port=3
  TestWaveOffsetRampEnd : Inport  Port=4
  TestWaveOffsetRampTime : Inport  Port=5
  TestWaveAmplitude : Inport  Port=6
  TestFreqRampStartFreq : Inport  Port=7
  TestFreqRampEndFreq : Inport  Port=8
  TestFreqRampTime : Inport  Port=9
  Enable : EnablePort  ZeroCross=off
  Constant2 : Constant  Value=ZERO
  Constant5 : Constant  Value=ZERO
  EdgeTriggered Pulse : $bdroot/Misc/EdgeTriggered Pulse  Edge=FALSE to TRUE  Width=single(0.01)  Pulse=TRUE  TimeStep=CLUTCH_INNER_LOOP_UPDATE_RATE  Init=0
  EdgeTriggered Pulse1 : $bdroot/Misc/EdgeTriggered Pulse  Edge=TRUE to FALSE  Width=single(0.01)  Pulse=TRUE  TimeStep=CLUTCH_INNER_LOOP_UPDATE_RATE  Init=0
  Logical Operator1 : Logic  Operator=OR  AllPortsSameDT=off
  Multiport Switch : MultiPortSwitch  DataPortOrder=Zero-based contiguous  Inputs=4  DataPortForDefault=Additional data port  zeroidx=on
  Switch2 : Switch  Threshold=0.5  ZeroCross=off
  TestFrequencyRamp : Subsystem
  TestOffsetRamp : Subsystem
  TestRampWaves : Subsystem
  TestWaveCreation : Subsystem
  Unit Delay1 : UnitDelay  InitialCondition=true  SampleTime=-1  HasFrameUpgradeWarning=on
      settings: AttributesFormatString=ic=%<X0>
  TestFreqRampFreq : Outport  InitialOutput=[single(0)]  VectorParamsAs1DForOutWhenUnconnected=off
      settings: AttributesFormatString=InitialOutput=%<InitialOutput>\nOutputWhenDisabled=%<OutputWhenDisabled>
  TestSignal : Outport  Port=2  InitialOutput=[single(0)]  VectorParamsAs1DForOutWhenUnconnected=off
      settings: AttributesFormatString=InitialOutput=%<InitialOutput>\nOutputWhenDisabled=%<OutputWhenDisabled>
  wires:
  TestOffsetRamp/2(TestOffsetRamp) -> TestRampWaves/1(TestOffsetRamp), Multiport Switch/3
  Constant5/1 -> Multiport Switch/6
  Multiport Switch/1 -> Switch2/1
  CluPresCmdTestSignalType/1 -> Multiport Switch/1, [CluPresCmdTestSignalType]
  Switch2/1 -> TestSignal/1  "TestSignal"
  Constant2/1 -> Switch2/3
  TestFrequencyRamp/1(TestFreqRampFreq) -> TestFreqRampFreq/1, TestWaveCreation/1(TestFreqRampFreq)
  Logical Operator1/1 -> Unit Delay1/1
  EdgeTriggered Pulse/1 -> Logical Operator1/1
  EdgeTriggered Pulse1/1 -> Logical Operator1/2
  TestSignalEnable/1 -> EdgeTriggered Pulse/1, EdgeTriggered Pulse1/1, [TestSignalEnable]
  Unit Delay1/1 -> [Test_Reset]
  [TestSignalEnable] -> TestFrequencyRamp/4(TestSignalEnable)
  TestFreqRampEndFreq/1 -> TestFrequencyRamp/2(TestFreqRampEndFreq)
  TestFreqRampStartFreq/1 -> TestFrequencyRamp/1(TestFreqRampStartFreq)
  TestFreqRampTime/1 -> TestFrequencyRamp/3(TestFreqRampTime)
  [Test_Reset] -> TestFrequencyRamp/5(Test_Reset)
  TestWaveAmplitude/1 -> TestWaveCreation/2(TestWaveAmplitude)
  [TestSignalEnable] -> TestOffsetRamp/4(Test_Enable)
  [Test_Reset] -> TestOffsetRamp/5(Test_Reset)
  TestWaveOffsetRampTime/1 -> TestOffsetRamp/3(TestWaveOffsetRampTime)
  TestWaveOffsetRampStart/1 -> TestOffsetRamp/1(TestWaveOffsetRampStart)
  TestWaveOffsetRampEnd/1 -> TestOffsetRamp/2(TestWaveOffsetRampEnd)
  TestOffsetRamp/1(TestConstant) -> Multiport Switch/2
  TestWaveCreation/1(TestWave) -> TestRampWaves/2(TestWave)
  [TestSignalEnable] -> Switch2/2
  [Test_Reset] -> TestWaveCreation/3(Test_Reset)
  [CluPresCmdTestSignalType] -> TestWaveCreation/4(CluPresCmdTestSignalType)
  TestWaveCreation/2(TestWaveSignSwitch) -> TestRampWaves/3(TestWaveSignSwitch)
  TestRampWaves/1(SineWave) -> Multiport Switch/4
  TestRampWaves/2(SquareWave) -> Multiport Switch/5

== system common_lib/Signal Generators/CustomProfileGenerator ==
  CustomProfileTimeVector : Inport
  CustomProfileOutputVector : Inport  Port=2
  CustomProfileRepeat : Inport  Port=3
  TestSignalReset : Inport  Port=4
  2D Lookup : $bdroot/Tbl/2D Lookup  Mode=Linear Interpolation
  Constant1 : Constant  Value=single(0.0)
  Logical Operator : Logic  Operator=OR  AllPortsSameDT=off
  Logical Operator1 : Logic  AllPortsSameDT=off
  MinMax : MinMax  Function=max  InputSameDT=on  ZeroCross=off
  Relational Operator : RelationalOperator  ZeroCross=off  RndMeth=Nearest
  Switch1 : Switch  Threshold=0.5  ZeroCross=off
  TestSignalTimer : $bdroot/Signal Generators/Signal Generator Components/TestSignalTimer  TimeStep=TimeStep
  Unit Delay5 : UnitDelay  InitialCondition=single(0.0)  SampleTime=-1  HasFrameUpgradeWarning=on
      settings: AttributesFormatString=ic=%<X0>
  CustomProfileOutput : Outport  VectorParamsAs1DForOutWhenUnconnected=off
  wires:
  TestSignalReset/1 -> [TestSignalReset], Logical Operator/1
  TestSignalTimer/1 -> [TestSignalTime]
  [TestSignalTime] -> 2D Lookup/1
  CustomProfileTimeVector/1 -> 2D Lookup/2, MinMax/1
  CustomProfileOutputVector/1 -> 2D Lookup/3
  MinMax/1 -> Relational Operator/2
  [TestSignalTime] -> Unit Delay5/1
  Unit Delay5/1 -> Relational Operator/1
  Relational Operator/1 -> Logical Operator1/2
  Logical Operator/1 -> TestSignalTimer/1
  CustomProfileRepeat/1 -> Logical Operator1/1
  Logical Operator1/1 -> Logical Operator/2
  Constant1/1 -> Switch1/1
  2D Lookup/1 -> Switch1/3
  [TestSignalReset] -> Switch1/2
  Switch1/1 -> CustomProfileOutput/1

== system common_lib/Signal Generators/Signal Generator Components ==
  note: Signal Generator Components
  TestSignalPeriod : Subsystem  mask{TimeStep=TimeStep}
      mask prompts: TimeStep "Time Step"
  TestSignalPeriodTimer : Subsystem  mask{TimeStep=TimeStep}
      mask prompts: TimeStep "Time Step"
  TestSignalRamp : Subsystem  mask{TimeStep=TimeStep}
      mask prompts: TimeStep "Time Step"
  TestSignalSineWave : Subsystem
  TestSignalSquareTriangleWave_Advanced : Subsystem  mask{TimeStep=TimeStep}
      mask prompts: TimeStep "Time Step"
  TestSignalSquareTriangleWave_Basic : Subsystem  mask{TimeStep=TimeStep}
      mask prompts: TimeStep "Time Step"
  TestSignalTimer : Subsystem  mask{TimeStep=TimeStep}
      mask prompts: TimeStep "Time Step"

== system common_lib/Signal Generators/SquareTriangleWaveDither ==
  CmdSignal : Inport
  CmdSignalMax : Inport  Port=2
  CmdSignalMin : Inport  Port=3
  DitherFrequency : Inport  Port=4
  DitherAmplitude : Inport  Port=5
  DitherOffset : Inport  Port=6
  DitherDutyCycle : Inport  Port=7
  DitherPhaseDelay : Inport  Port=8
  DitherOffsetRatio : Inport  Port=9
  DitherTri2SqRatio : Inport  Port=10
  DitherReset : Inport  Port=11
  Constant : Constant  Value=single(1)  SampleTime=-1
  MinMax : MinMax  Inputs=2  InputSameDT=on  ZeroCross=off
  Product1 : Product  OutDataTypeStr=Inherit: Same as first input
  Sat : $bdroot/Slink/Sat
  SquareTriangleWaveGenerator_Advanced : $bdroot/Signal Generators/SquareTriangleWaveGenerator_Advanced  TimeStep=TimeStep
  Dither : Outport  VectorParamsAs1DForOutWhenUnconnected=off
  wires:
  Constant/1 -> Product1/2
  Product1/1 -> SquareTriangleWaveGenerator_Advanced/2
  MinMax/1 -> Product1/1
  Sat/1 -> MinMax/1
  CmdSignalMax/1 -> Sat/2
  CmdSignalMin/1 -> Sat/3
  SquareTriangleWaveGenerator_Advanced/1 -> Dither/1
  CmdSignal/1 -> Sat/1
  DitherReset/1 -> SquareTriangleWaveGenerator_Advanced/8
  DitherTri2SqRatio/1 -> SquareTriangleWaveGenerator_Advanced/7
  DitherOffsetRatio/1 -> SquareTriangleWaveGenerator_Advanced/6
  DitherPhaseDelay/1 -> SquareTriangleWaveGenerator_Advanced/5
  DitherDutyCycle/1 -> SquareTriangleWaveGenerator_Advanced/4
  DitherOffset/1 -> SquareTriangleWaveGenerator_Advanced/3
  DitherAmplitude/1 -> MinMax/2
  DitherFrequency/1 -> SquareTriangleWaveGenerator_Advanced/1

== system common_lib/Signal Generators/SquareTriangleWaveDitherPWM ==
  note: Output Type:
      | 0 - Dither
      | 1 - PWM
  CmdSignal : Inport
  OutputType : Inport  Port=2
  CmdSignalMax : Inport  Port=3
  CmdSignalMin : Inport  Port=4
  DitherFrequency : Inport  Port=5
  DitherAmplitude : Inport  Port=6
  DitherOffset : Inport  Port=7
  DitherDutyCycle : Inport  Port=8
  DitherPhaseDelay : Inport  Port=9
  DitherOffsetRatio : Inport  Port=10
  DitherTri2SqRatio : Inport  Port=11
  DitherReset : Inport  Port=12
  Constant : Constant  Value=single(1)  SampleTime=-1
  MinMax : MinMax  Inputs=2  InputSameDT=on  ZeroCross=off
  Product1 : Product  OutDataTypeStr=Inherit: Same as first input
  Sat : $bdroot/Slink/Sat
  SquareTriangleWaveGenerator_Advanced : $bdroot/Signal Generators/SquareTriangleWaveGenerator_Advanced  TimeStep=TimeStep
  Switch : Switch  Threshold=0.5  ZeroCross=off
  Dither_PWM : Outport  VectorParamsAs1DForOutWhenUnconnected=off
  wires:
  Constant/1 -> Product1/2
  Product1/1 -> Switch/3
  MinMax/1 -> Product1/1
  Sat/1 -> MinMax/2
  CmdSignalMax/1 -> Sat/2
  CmdSignalMin/1 -> Sat/3
  CmdSignal/1 -> Sat/1
  DitherReset/1 -> SquareTriangleWaveGenerator_Advanced/8
  DitherTri2SqRatio/1 -> SquareTriangleWaveGenerator_Advanced/7
  DitherOffsetRatio/1 -> SquareTriangleWaveGenerator_Advanced/6
  DitherPhaseDelay/1 -> SquareTriangleWaveGenerator_Advanced/5
  DitherOffset/1 -> SquareTriangleWaveGenerator_Advanced/3
  DitherAmplitude/1 -> MinMax/1, Switch/1
  DitherFrequency/1 -> SquareTriangleWaveGenerator_Advanced/1
  OutputType/1 -> Switch/2
  SquareTriangleWaveGenerator_Advanced/1 -> Dither_PWM/1  "Dither_PWM"
  Switch/1 -> SquareTriangleWaveGenerator_Advanced/2
  DitherDutyCycle/1 -> SquareTriangleWaveGenerator_Advanced/4

== system common_lib/Signal Generators/SquareTriangleWaveGenerator_Advanced ==
  TestSignalFrequency : Inport
  TestSignalPk2PkAmplitude : Inport  Port=2
  TestSignalOffset : Inport  Port=3
  TestSignalDutyCycle : Inport  Port=4
  TestSignalPhaseDelay : Inport  Port=5
  TestSignalOffsetRatio : Inport  Port=6
  TestSignalTri2SqRatio : Inport  Port=7
  TestSignalReset : Inport  Port=8
  TestSignalPeriod : $bdroot/Signal Generators/Signal Generator Components/TestSignalPeriod  TimeStep=TimeStep
  TestSignalPeriodTimer : $bdroot/Signal Generators/Signal Generator Components/TestSignalPeriodTimer  TimeStep=TimeStep
  TestSignalSquareTriangleWave_Advanced : $bdroot/Signal Generators/Signal Generator Components/TestSignalSquareTriangleWave_Advanced  TimeStep=TimeStep
  TestSignal : Outport  VectorParamsAs1DForOutWhenUnconnected=off
  wires:
  [TestSignalReset] -> TestSignalSquareTriangleWave_Advanced/9
  TestSignalTri2SqRatio/1 -> TestSignalSquareTriangleWave_Advanced/8
  TestSignalSquareTriangleWave_Advanced/1 -> TestSignal/1
  TestSignalPk2PkAmplitude/1 -> TestSignalSquareTriangleWave_Advanced/3
  TestSignalFrequency/1 -> TestSignalPeriod/1
  TestSignalPeriod/1 -> TestSignalSquareTriangleWave_Advanced/2, TestSignalPeriodTimer/2
  TestSignalReset/1 -> [TestSignalReset], TestSignalPeriodTimer/1
  TestSignalOffset/1 -> TestSignalSquareTriangleWave_Advanced/4
  TestSignalPeriodTimer/1 -> TestSignalSquareTriangleWave_Advanced/1
  TestSignalDutyCycle/1 -> TestSignalSquareTriangleWave_Advanced/5
  TestSignalPhaseDelay/1 -> TestSignalSquareTriangleWave_Advanced/6
  TestSignalOffsetRatio/1 -> TestSignalSquareTriangleWave_Advanced/7

== system common_lib/Signal Generators/SquareTriangleWaveGenerator_Basic ==
  TestSignalFrequency : Inport
  TestSignalPk2PkAmplitude : Inport  Port=2
  TestSignalOffset : Inport  Port=3
  TestSignalTri2SqRatio : Inport  Port=4
  TestSignalReset : Inport  Port=5
  TestSignalPeriod : $bdroot/Signal Generators/Signal Generator Components/TestSignalPeriod  TimeStep=TimeStep
  TestSignalPeriodTimer : $bdroot/Signal Generators/Signal Generator Components/TestSignalPeriodTimer  TimeStep=TimeStep
  TestSignalSquareTriangleWave_Basic : $bdroot/Signal Generators/Signal Generator Components/TestSignalSquareTriangleWave_Basic  TimeStep=TimeStep
  TestSignal : Outport  VectorParamsAs1DForOutWhenUnconnected=off
  wires:
  [TestSignalReset] -> TestSignalSquareTriangleWave_Basic/6
  TestSignalTri2SqRatio/1 -> TestSignalSquareTriangleWave_Basic/5
  TestSignalSquareTriangleWave_Basic/1 -> TestSignal/1
  TestSignalPk2PkAmplitude/1 -> TestSignalSquareTriangleWave_Basic/3
  TestSignalFrequency/1 -> TestSignalPeriod/1
  TestSignalPeriod/1 -> TestSignalSquareTriangleWave_Basic/2, TestSignalPeriodTimer/2
  TestSignalReset/1 -> [TestSignalReset], TestSignalPeriodTimer/1
  TestSignalOffset/1 -> TestSignalSquareTriangleWave_Basic/4
  TestSignalPeriodTimer/1 -> TestSignalSquareTriangleWave_Basic/1

== system common_lib/Signal Routing/Overwrite ==
  In1 : Inport
  Data Type Conversion : DataTypeConversion  OutDataTypeStr=single
  Data Type Conversion1 : DataTypeConversion  OutDataTypeStr=single
  Switch : Switch  Threshold=0.5
  xPCOE_VariableName : Constant  Value=OverwriteEnable
  xPCOV_VariableName : Constant  Value=OverwriteValue
  Out1 : Outport  VectorParamsAs1DForOutWhenUnconnected=off
  wires:
  Switch/1 -> Out1/1
  xPCOE_VariableName/1 -> Data Type Conversion1/1
  xPCOV_VariableName/1 -> Data Type Conversion/1
  In1/1 -> Switch/3
  Data Type Conversion/1 -> Switch/1
  Data Type Conversion1/1 -> Switch/2

== system common_lib/Signal Routing/Vector to Bus ==
  VectorIn : Inport
  Bus Creator3 : BusCreator  Inputs=8
  Demux : Demux  Outputs=8
  BusOut : Outport  VectorParamsAs1DForOutWhenUnconnected=off
  wires:
  Demux/1 -> Bus Creator3/1  "output_driver_enable"
  Demux/2 -> Bus Creator3/2  "shft_cyl_12_Icmd"
  Demux/3 -> Bus Creator3/3  "shft_cyl_R_Icmd"
  Demux/4 -> Bus Creator3/4  "shft_cyl_3_Icmd"
  Bus Creator3/1 -> BusOut/1
  VectorIn/1 -> Demux/1
  Demux/5 -> Bus Creator3/5  "shft_cyl_5_Icmd"
  Demux/6 -> Bus Creator3/6  "shft_cyl_4_Icmd"
  Demux/7 -> Bus Creator3/7  "shft_cyl_6_Icmd"
  Demux/8 -> Bus Creator3/8  "shft_cyl_UL_Icmd"

== system common_lib/Slink/Dead ==
  note: This is a soft deadband block.
      |
      |    If the absolute value of the Input is less than the deadband, the Output is zero
      | Otherwise, the output smoothly increases outside the deadband,
      |    thereby providing smooth transition in and out of the deadband.
  note: Common Library::Simulink Enhancements::Deadband
  input : Inport
  deadband : Inport  Port=2
  Constant1 : Constant  Value=Zero
  Constant2 : Constant  Value=MinusOne
  R1 : Sum  Inputs=+-  InputSameDT=on  OutDataTypeStr=Inherit: Same as first input
  R2 : Sum  Inputs=+-  InputSameDT=on  OutDataTypeStr=Inherit: Same as first input
  Relational Operator6 : RelationalOperator  ZeroCross=off  RndMeth=Nearest  InputSameDT=on
  Relational Operator7 : RelationalOperator  Operator=>  ZeroCross=off  RndMeth=Nearest  InputSameDT=on
  Switch2 : Switch  Threshold=0.5  ZeroCross=off  InputSameDT=on
  Switch3 : Switch  Threshold=0.5  ZeroCross=off  InputSameDT=on
  mep to torque2 : Product  InputSameDT=on  OutDataTypeStr=Inherit: Same as first input
  output : Outport  VectorParamsAs1DForOutWhenUnconnected=off
  wires:
  Constant2/1 -> mep to torque2/2
  Switch2/1 -> output/1
  Constant1/1 -> Switch3/1
  Switch3/1 -> Switch2/3
  R2/1 -> Switch3/3
  Relational Operator6/1 -> Switch3/2
  R1/1 -> Switch2/1
  Relational Operator7/1 -> Switch2/2
  mep to torque2/1 -> R2/2, Relational Operator6/2
  deadband/1 -> Relational Operator7/2, R1/2, mep to torque2/1
  input/1 -> R1/1, Relational Operator6/1, R2/1, Relational Operator7/1

== system common_lib/Slink/Hysteresis ==
  note: Common Library::Simulink Enhancements::Hysteresis
  Input : Inport
  Delta : Inport  Port=2
  Constant4 : Constant  Value=MinusOne
  Product1 : Product  InputSameDT=on  OutDataTypeStr=Inherit: Same as first input
  Sat : $bdroot/Slink/Sat
  Sum : Sum  Inputs=+-+  InputSameDT=on  OutDataTypeStr=Inherit: Same as first input
  Sum2 : Sum  Inputs=+-  InputSameDT=on  OutDataTypeStr=Inherit: Same as first input
  Unit Delay1 : UnitDelay  InitialCondition=IC  SampleTime=-1  HasFrameUpgradeWarning=on
  Unit Delay2 : UnitDelay  InitialCondition=IC  SampleTime=-1  HasFrameUpgradeWarning=on
  Output : Outport  VectorParamsAs1DForOutWhenUnconnected=off
  wires:
  Input/1 -> Unit Delay2/1, Sum/1, Sum2/1
  Constant4/1 -> Product1/2
  Unit Delay2/1 -> Sum/2
  Delta/1 -> Sat/2, Product1/1
  Product1/1 -> Sat/3
  Sum/1 -> Sat/1
  Sat/1 -> Sum2/2, Unit Delay1/1
  Sum2/1 -> Output/1
  Unit Delay1/1 -> Sum/3

== system common_lib/Slink/Relay ==
  note: Common Library::Simulink Enhancements::Relay
  input : Inport
  upper_thd : Inport  Port=2
  lower_thd : Inport  Port=3
  upper_value : Inport  Port=4
  lower_value : Inport  Port=5
  Relational Operator1 : RelationalOperator  Operator=<=  ZeroCross=off  RndMeth=Nearest  InputSameDT=on
  Relational Operator7 : RelationalOperator  ZeroCross=off  RndMeth=Nearest  InputSameDT=on
  Switch1 : Switch  Threshold=0.5  ZeroCross=off  InputSameDT=on
  Switch3 : Switch  Threshold=0.5  ZeroCross=off  InputSameDT=on
  Unit Delay : UnitDelay  InitialCondition=init  SampleTime=-1  HasFrameUpgradeWarning=on
  output : Outport  VectorParamsAs1DForOutWhenUnconnected=off
  wires:
  Switch3/1 -> Unit Delay/1, output/1
  Switch1/1 -> Switch3/3
  Unit Delay/1 -> Switch1/3
  Relational Operator1/1 -> Switch1/2
  lower_value/1 -> Switch1/1
  Relational Operator7/1 -> Switch3/2
  upper_value/1 -> Switch3/1
  lower_thd/1 -> Relational Operator1/2
  input/1 -> Relational Operator1/1, Relational Operator7/1
  upper_thd/1 -> Relational Operator7/2

== system common_lib/Slink/Relay_1 ==
  note: Common Library::Simulink Enhancements::Relay
  input : Inport
  Delta : Inport  Port=2
  B : Inport  Port=3
  Relational Operator7 : RelationalOperator  Operator=<=  ZeroCross=off  RndMeth=Nearest  InputSameDT=on
  Sum : Sum
  Switch3 : Switch  Threshold=0.5  ZeroCross=off  InputSameDT=on
  output : Outport  VectorParamsAs1DForOutWhenUnconnected=off
  wires:
  Sum/1 -> Relational Operator7/2
  Delta/1 -> Sum/1
  Switch3/1 -> output/1
  Relational Operator7/1 -> Switch3/2
  B/1 -> Relational Operator7/1, Switch3/1
  input/1 -> Sum/2, Switch3/3

== system common_lib/Slink/Sat ==
  note: Common Library::Simulink Enhancements::Saturation
  input : Inport
  ulim : Inport  Port=2
  llim : Inport  Port=3
  MinMax : MinMax  Function=max  Inputs=2  InputSameDT=on  ZeroCross=off
  MinMax1 : MinMax  Inputs=2  InputSameDT=on  ZeroCross=off
  output : Outport  VectorParamsAs1DForOutWhenUnconnected=off
  wires:
  MinMax/1 -> output/1
  llim/1 -> MinMax/2
  MinMax1/1 -> MinMax/1
  ulim/1 -> MinMax1/2
  input/1 -> MinMax1/1

== system common_lib/Slink/Three Value Threshold ==
  note: Common Library::Simulink Enhancements::
  input : Inport
  upper_thd : Inport  Port=2
  lower_thd : Inport  Port=3
  upper_value : Inport  Port=4
  relay_value : Inport  Port=5
  lower_value : Inport  Port=6
  Relational Operator1 : RelationalOperator  Operator=<=  ZeroCross=off  RndMeth=Nearest  InputSameDT=on
  Relational Operator7 : RelationalOperator  ZeroCross=off  RndMeth=Nearest  InputSameDT=on
  Switch1 : Switch  Threshold=0.5  ZeroCross=off  InputSameDT=on
  Switch3 : Switch  Threshold=0.5  ZeroCross=off  InputSameDT=on
  output : Outport  VectorParamsAs1DForOutWhenUnconnected=off
  wires:
  relay_value/1 -> Switch1/3
  upper_thd/1 -> Relational Operator7/2
  input/1 -> Relational Operator7/1, Relational Operator1/1
  lower_thd/1 -> Relational Operator1/2
  upper_value/1 -> Switch3/1
  Relational Operator7/1 -> Switch3/2
  lower_value/1 -> Switch1/1
  Relational Operator1/1 -> Switch1/2
  Switch1/1 -> Switch3/3
  Switch3/1 -> output/1
